simulink model "QAM_passmodem"  (Simulink 8.7)
settings: Solver=FixedStepDiscrete  SolverMode=SingleTasking  StartTime=0.0  StopTime=2  FixedStep=1/100000  RelTol=1e-3  AbsTol=1e-6
PreLoadFcn:
  | fs=1e5; Ts=1/fs; R=1000; T=1/R; fc=10000; M=16; A=1;
libraries: commfilt2 x2, commchan3 x1, commrandsrc2 x1
settings Model: Creator=amoura  LastModifiedBy=Artur Moura
settings DataIOCC: LimitDataPoints=off  SignalLoggingSaveFormat=ModelDataLogs
settings OptimizationCC: BlockReduction=off  BooleanDataType=off  ExpressionDepthLimit=2147483647  InitFltsAndDblsToZero=on
settings DebuggingCC: SaveWithParameterizedLinksMsg=none  SignalResolutionControl=TryResolveAllWithWarning  MultiTaskDSMMsg=warning  MultiTaskCondExecSysMsg=none  FcnCallInpInsideContextMsg=UseLocalSettings  StateNameClashWarn=warning
settings HardwareCC: TargetUnknown=on
settings RTWCC: TemplateMakefile=grt_unix.tmf
settings GRTTargetCC: TargetFcnLib=ansi_tfl_tmw.mat  ModelReferenceCompliant=off  CombineOutputUpdateFcns=off  MatFileLogging=off  GRTInterface=on

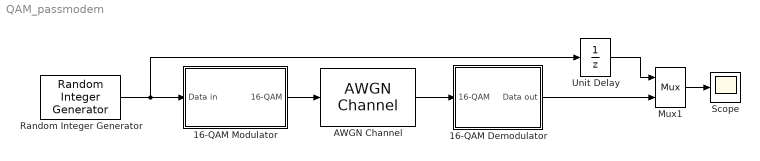
== system QAM_passmodem ==
  16-QAM Demodulator : Subsystem
  16-QAM Modulator : Subsystem
  AWGN Channel : commchan3/AWGN Channel  InputProcessing=Columns as channels (frame based)  seed=67  noiseMode="Signal to noise ratio  (Es/No)"  EbNodB=0  EsNodB=16  SNRdB=10  bitsPerSym=1  Ps=1  Tsym=T  variance=1
  Mux1 : Mux  Inputs=2
  Random Integer Generator : commrandsrc2/Random Integer Generator  mul=M  seed=529558  Ts=T  frameBased=off  sampPerFrame=100  orient=off  outDataType=double
  Scope : Scope
  Unit Delay : UnitDelay  SampleTime=1/1000
  wires:
  16-QAM Modulator/1(16-QAM) -> AWGN Channel/1
  Unit Delay/1 -> Mux1/1
  Mux1/1 -> Scope/1
  Random Integer Generator/1 -> Unit Delay/1, 16-QAM Modulator/1(Data in)
  16-QAM Demodulator/1(Data out) -> Mux1/2
  AWGN Channel/1 -> 16-QAM Demodulator/1(16-QAM)

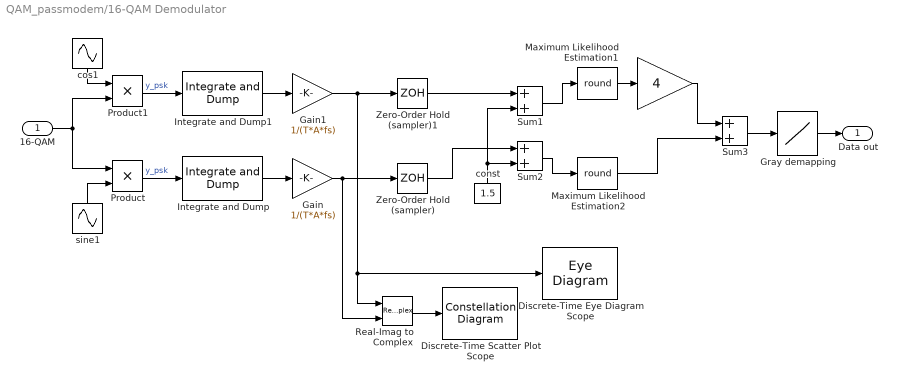
== system QAM_passmodem/16-QAM Demodulator ==
  16-QAM : Inport
  "  " : Gain  Gain=4  SaturateOnIntegerOverflow=on  OutDataTypeStr=Inherit: Same as input  ParamDataTypeStr=Inherit: Same as input
  Discrete-Time Eye Diagram Scope : EyeDiagram  Tag=EyeDiagram
  Discrete-Time Scatter Plot Scope : ConstellationDiagram  Tag=ScatterPlot
  Gain : Gain  Gain=1/(T*A*fs)  SampleTime=Ts  SaturateOnIntegerOverflow=on  OutDataTypeStr=Inherit: Same as input  ParamDataTypeStr=Inherit: Same as input
  Gain1 : Gain  Gain=1/(T*A*fs)  SampleTime=Ts  SaturateOnIntegerOverflow=on  OutDataTypeStr=Inherit: Same as input  ParamDataTypeStr=Inherit: Same as input
  Gray demapping : Lookup_n-D  NumberOfTableDimensions=1  BreakpointsForDimension1=[0 1 2 3 4 5 6 7 8 9 10 11 12 13 14 15]  Table=[4 12 8 0 5 13 9 1 7 15 11 3 6 14 10 2]  SaturateOnIntegerOverflow=on  InputSameDT=on
  Integrate and Dump : commfilt2/Integrate and Dump  obssamples=T/Ts  offsetsamples=1  nodump=on  roundingMode=Floor  overflowMode=off  outputDataTypeStr=Inherit: Same as accumulator  outputLastDataTypeStr=Inherit: Same as accumulator
  Integrate and Dump1 : commfilt2/Integrate and Dump  obssamples=T/Ts  offsetsamples=1  nodump=on  roundingMode=Floor  overflowMode=off  outputDataTypeStr=Inherit: Same as accumulator  outputLastDataTypeStr=Inherit: Same as accumulator
  Maximum Likelihood Estimation1 : Rounding  Operator=round
  Maximum Likelihood Estimation2 : Rounding  Operator=round
  Product : Product  SampleTime=1/100000  SaturateOnIntegerOverflow=on  RndMeth=Zero  InputSameDT=on  OutDataTypeStr=Inherit: Same as first input
  Product1 : Product  SampleTime=1/100000  SaturateOnIntegerOverflow=on  RndMeth=Zero  InputSameDT=on  OutDataTypeStr=Inherit: Same as first input
  Real-Imag to Complex : RealImagToComplex
  Sum1 : Sum  SaturateOnIntegerOverflow=on  InputSameDT=on  OutDataTypeStr=Inherit: Same as first input
  Sum2 : Sum  SaturateOnIntegerOverflow=on  InputSameDT=on  OutDataTypeStr=Inherit: Same as first input
  Sum3 : Sum  SaturateOnIntegerOverflow=on  InputSameDT=on  OutDataTypeStr=Inherit: Same as first input
  Zero-Order Hold (sampler) : ZeroOrderHold  SampleTime=1/1000
  Zero-Order Hold (sampler)1 : ZeroOrderHold  SampleTime=1/1000
  const : Constant  Value=1.5
  cos1 : Sin  Frequency=2*pi*fc  Phase=pi/2  SampleTime=0
  sine1 : Sin  Frequency=2*pi*fc  SampleTime=0
  Data out : Outport
  wires:
  Product/1 -> Integrate and Dump/1  "y_psk"
  16-QAM/1 -> Product1/2, Product/1
  Integrate and Dump/1 -> Gain/1
  sine1/1 -> Product/2
  Product1/1 -> Integrate and Dump1/1  "y_psk"
  Integrate and Dump1/1 -> Gain1/1
  cos1/1 -> Product1/1
  Gain1/1 -> Zero-Order Hold (sampler)1/1, Discrete-Time Eye Diagram Scope/1, Real-Imag to Complex/1
  Gain/1 -> Zero-Order Hold (sampler)/1, Real-Imag to Complex/2
  "  "/1 -> Sum3/1
  Sum3/1 -> Gray demapping/1
  const/1 -> Sum1/2, Sum2/2
  Sum1/1 -> Maximum Likelihood Estimation1/1
  Sum2/1 -> Maximum Likelihood Estimation2/1
  Zero-Order Hold (sampler)1/1 -> Sum1/1
  Maximum Likelihood Estimation1/1 -> "  "/1
  Maximum Likelihood Estimation2/1 -> Sum3/2
  Zero-Order Hold (sampler)/1 -> Sum2/1
  Real-Imag to Complex/1 -> Discrete-Time Scatter Plot Scope/1
  Gray demapping/1 -> Data out/1

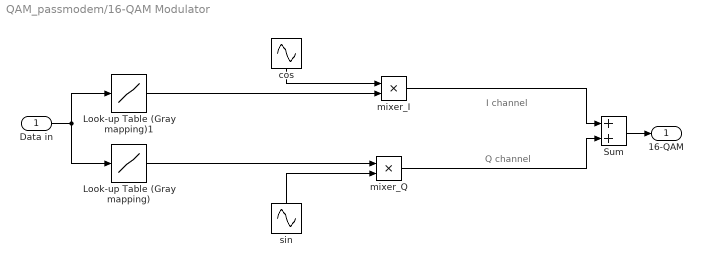
== system QAM_passmodem/16-QAM Modulator ==
  note: I channel
  note: Q channel
  Data in : Inport
  Look-up Table (Gray mapping) : Lookup_n-D  NumberOfTableDimensions=1  BreakpointsForDimension1=[0 1 2 3 4 5 6 7 8 9 10 11 12 13 14 15]  Table=[3*A 3*A 3*A 3*A -3*A -3*A -3*A -3*A A A A A -A -A -A -A ]  SaturateOnIntegerOverflow=on  InputSameDT=on
  Look-up Table (Gray mapping)1 : Lookup_n-D  NumberOfTableDimensions=1  BreakpointsForDimension1=[0 1 2 3 4 5 6 7 8 9 10 11 12 13 14 15]  Table=[-3*A -A 3*A A -3*A -A 3*A A -3*A -A 3*A A -3*A -A 3*A A]  SaturateOnIntegerOverflow=on  InputSameDT=on
  Sum : Sum  SaturateOnIntegerOverflow=on  InputSameDT=on  OutDataTypeStr=Inherit: Same as first input
  cos : Sin  Frequency=2*pi*fc  Phase=pi/2  SampleTime=0
  mixer_I : Product  SaturateOnIntegerOverflow=on  InputSameDT=on  OutDataTypeStr=Inherit: Same as first input
  mixer_Q : Product  SaturateOnIntegerOverflow=on  InputSameDT=on  OutDataTypeStr=Inherit: Same as first input
  sin : Sin  Frequency=2*pi*fc  SampleTime=0
  16-QAM : Outport
  wires:
  Look-up Table (Gray mapping)1/1 -> mixer_I/2
  Data in/1 -> Look-up Table (Gray mapping)1/1, Look-up Table (Gray mapping)/1
  mixer_I/1 -> Sum/1
  mixer_Q/1 -> Sum/2
  sin/1 -> mixer_Q/2
  cos/1 -> mixer_I/1
  Sum/1 -> 16-QAM/1
  Look-up Table (Gray mapping)/1 -> mixer_Q/1
